simulink model "ExtremumSeekingControl_example"  (R2022b)
settings: Solver=VariableStepAuto  StartTime=0.0  StopTime=15  RelTol=1e-3
settings Model: Creator=The MathWorks, Inc.  LastModifiedBy=Claudia Yasar
settings DataIOCC: ReturnWorkspaceOutputs=off
settings DebuggingCC: UnconnectedInputMsg=warning  UnconnectedOutputMsg=warning  UnconnectedLineMsg=warning
settings ModelReferenceCC: EnableRefExpFcnMdlSchedulingChecks=on
settings RTWCC: DLArmComputeVersion=19.05

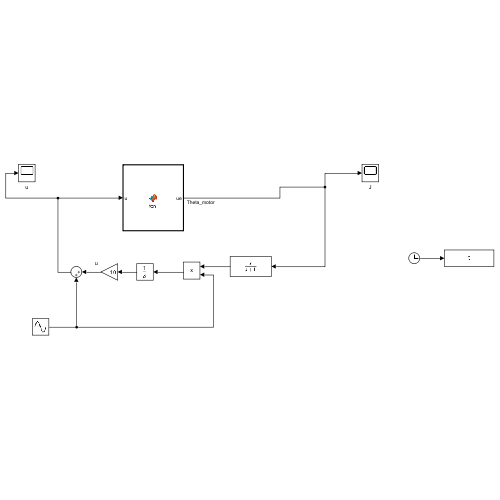
[thumbnail: Simulink's stored preview of the top-level diagram]
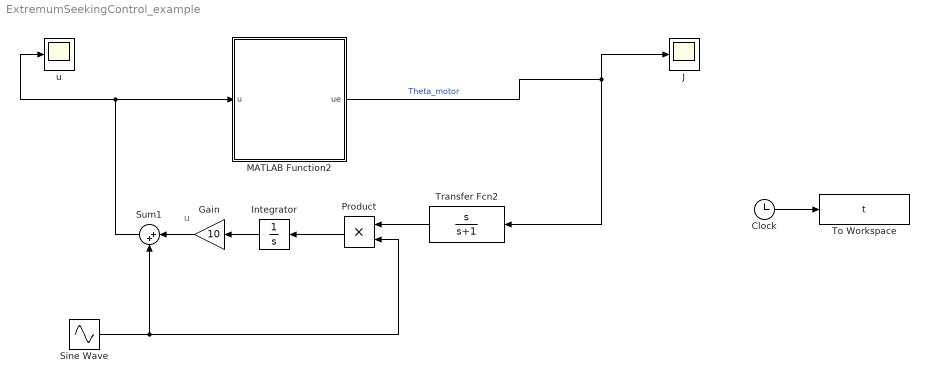
== system ExtremumSeekingControl_example ==
  note: u
  Clock : Clock
  Gain : Gain  Gain=10
  Integrator : Integrator
  J : Scope
  MATLAB Function2 : MATLAB Function  TreatAsAtomicUnit=on
  Product : Product
  Sine Wave : Sin  Amplitude=0.5  Frequency=2*pi*10  SampleTime=0
  Sum1 : Sum  Inputs=|++
  To Workspace : ToWorkspace  VariableName=t  SaveFormat=Timeseries  SampleTime=-1
  Transfer Fcn2 : TransferFcn  Numerator=[1 0]  Denominator="[1  1]"
  u : Scope
  wires:
  Clock/1 -> To Workspace/1
  Sum1/1 -> u/1, MATLAB Function2/1(u)
  Integrator/1 -> Gain/1
  Product/1 -> Integrator/1
  Gain/1 -> Sum1/1
  Sine Wave/1 -> Product/2, Sum1/2
  MATLAB Function2/1(ue) -> Transfer Fcn2/1, J/1  "Theta_motor"
  Transfer Fcn2/1 -> Product/1

== matlab function ExtremumSeekingControl_example/MATLAB Function2 ==
  data: u input; ue output
function ue = fcn(u)



ue = 25-(5-u)^2;
